simulink model "nxtmouse_ctrl"  (Simulink 6.4)
settings: Solver=FixedStepDiscrete  SolverMode=SingleTasking  StartTime=0  StopTime=inf  FixedStep=0.001  RelTol=1e-3
PreLoadFcn:
  | param;
libraries: ecrobot_nxt_lib x13
CloseFcn:
  | rtwprivate ssgencode ModelCloseRequest nxtcar_ctrl
settings Model: Creator=tchikama  LastModifiedBy=tchikama  ProdHWDeviceType=ARM7
settings DataIOCC: LimitDataPoints=off  SaveOutput=off  SignalLogging=off  SaveTime=off
settings OptimizationCC: InlineParams=on  InlineInvariantSignals=on  RollThreshold=2  StateBitsets=on  DataBitsets=on  UseTempVars=on  InitFltsAndDblsToZero=off  NoFixptDivByZeroProtection=on  EfficientFloat2IntCast=on  OptimizeModelRefInitCode=on  LifeSpan=1
settings DebuggingCC: ConsistencyChecking=warning  SignalInfNanChecking=warning  ReadBeforeWriteMsg=DisableAll  WriteAfterWriteMsg=DisableAll  WriteAfterReadMsg=DisableAll  AlgebraicLoopMsg=error  CheckExecutionContextPreStartOutputMsg=on  CheckExecutionContextRuntimeOutputMsg=on  SolverPrmCheckMsg=none  SingleTaskRateTransMsg=warning  TasksWithSamePriorityMsg=none  IntegerOverflowMsg=error  ParameterUnderflowMsg=warning  ParameterPrecisionLossMsg=none  UnconnectedInputMsg=error  UnconnectedOutputMsg=error  UnconnectedLineMsg=error  UniqueDataStoreMsg=error  BusObjectLabelMismatch=error  RootOutportRequireBusObject=error  ModelReferenceIOMsg=warning  ModelReferenceVersionMismatchMessage=warning  ModelReferenceIOMismatchMessage=warning
settings HardwareCC: ProdIntDivRoundTo=Zero  ProdEndianess=LittleEndian  ProdHWDeviceType=ARM7  TargetHWDeviceType=32-bit Generic
settings ModelReferenceCC: ModelReferenceNumInstancesAllowed=Single
settings RTWCC: SystemTargetFile=ert.tlc  GenCodeOnly=on  GenerateMakefile=off  TemplateMakefile=ert_default_tmf  Description=Real-Time Workshop Embedded Coder (no auto configuration)  GenerateReport=on  RTWVerbose=off  ProcessScript=ert_make_rtw_hook  IncludeHyperlinkInReport=on  LaunchReport=on
settings CodeAppCC: ForceParamTrailComments=on  IgnoreCustomStorageClasses=off  SFDataObjDesc=on  PrefixModelToSubsysFcnNames=off  CustomSymbolStrGlobalVar=rt$N$M  CustomSymbolStrType=$N$M  CustomSymbolStrFcn=$N$M$F  CustomSymbolStrMacro=$N$M  InsertBlockDesc=on
settings ERTTargetCC: TargetFcnLib=ansi_tfl_tmw.mat  GenFloatMathFcnCalls=GNU  IncludeMdlTerminateFcn=off  SuppressErrorStatus=on  IncludeERTFirstTime=on  SupportAbsoluteTime=off  SupportNonFinite=off  SupportComplex=off  PurelyIntegerCode=on  InlinedParameterPlacement=NonHierarchical  RootIOFormat=Structure reference  ERTCustomFileTemplate=example_file_process.tlc  InitialValueSource=Model

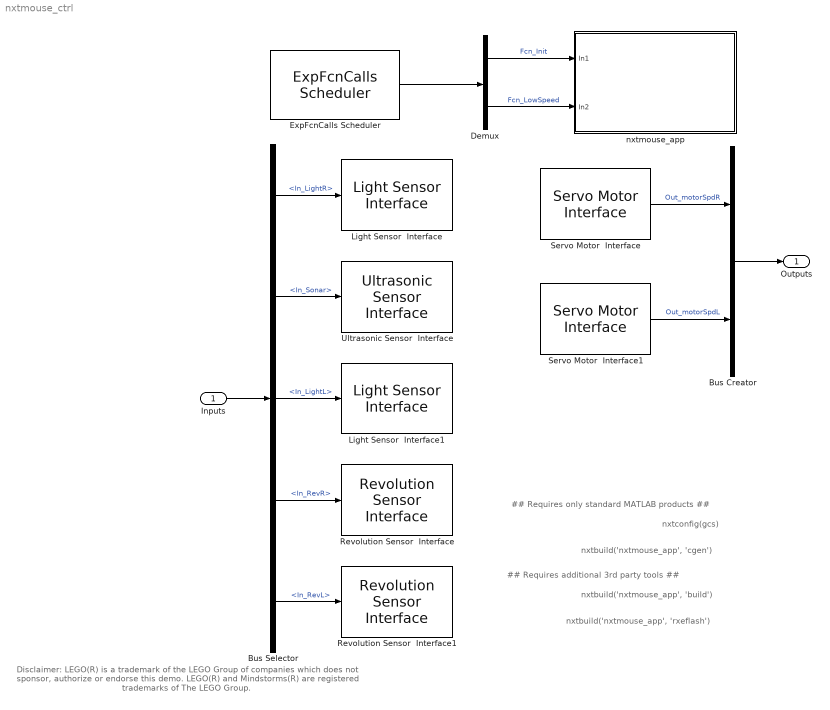
== system nxtmouse_ctrl ==
  note: nxtbuild('nxtmouse_app', 'cgen')
  note: nxtconfig(gcs)
  note: Disclaimer:
      | LEGO(R) is a trademark of the LEGO Group of companies which does not sponsor, authorize or endorse this demo.
      | LEGO(R) and Mindstorms(R)  are registered trademarks of The LEGO Group.
  note: nxtbuild('nxtmouse_app', 'build')
  note: nxtbuild('nxtmouse_app', 'rxeflash')
  note: ## Requires only standard MATLAB products ##
  note: ## Requires additional 3rd party tools ##
  Inputs : Inport  UseBusObject=on
      settings: BusObject=Inputs
  Bus Creator : BusCreator  Inputs=2  UseBusObject=on
      settings: BusObject=Outputs
  Bus Selector : BusSelector  OutputSignals=In_LightR,In_Sonar,In_LightL,In_RevR,In_RevL
  Demux : Demux  Outputs=2
  ExpFcnCalls Scheduler : ecrobot_nxt_lib/ExpFcnCalls Scheduler  Priority=50  fcname='Fcn_Init', 'Fcn_LowSpeed'  fctrigger=[0 50]  ts=0.001  platform=OSEK  stacksize=[512 512]  bd_mode=Slave
  Light Sensor  Interface : ecrobot_nxt_lib/Light Sensor Interface  Priority=0  SystemSampleTime=-1  ip=S2
  Light Sensor  Interface1 : ecrobot_nxt_lib/Light Sensor Interface  Priority=2  SystemSampleTime=-1  ip=S3
  Revolution Sensor  Interface : ecrobot_nxt_lib/Revolution Sensor Interface  Priority=3  SystemSampleTime=-1  ip=B
  Revolution Sensor  Interface1 : ecrobot_nxt_lib/Revolution Sensor Interface  Priority=4  SystemSampleTime=-1  ip=C
  Servo Motor  Interface : ecrobot_nxt_lib/Servo Motor Interface  Priority=100  SystemSampleTime=-1  ip=B  mode=Brake
  Servo Motor  Interface1 : ecrobot_nxt_lib/Servo Motor Interface  Priority=101  SystemSampleTime=-1  ip=C  mode=Brake
  Ultrasonic Sensor  Interface : ecrobot_nxt_lib/Ultrasonic Sensor Interface  Priority=1  SystemSampleTime=-1  ip=S1
  nxtmouse_app : Subsystem
  Outputs : Outport  UseBusObject=on
      settings: BusObject=Outputs
  wires:
  Bus Selector/4 -> Revolution Sensor  Interface/1  "<In_RevR>"
  Bus Selector/5 -> Revolution Sensor  Interface1/1  "<In_RevL>"
  Bus Creator/1 -> Outputs/1
  Inputs/1 -> Bus Selector/1
  Servo Motor  Interface/1 -> Bus Creator/1  "Out_motorSpdR"
  Servo Motor  Interface1/1 -> Bus Creator/2  "Out_motorSpdL"
  ExpFcnCalls Scheduler/1 -> Demux/1
  Demux/1 -> nxtmouse_app/1(In1)  "Fcn_Init"
  Demux/2 -> nxtmouse_app/2(In2)  "Fcn_LowSpeed"
  Bus Selector/2 -> Ultrasonic Sensor  Interface/1  "<In_Sonar>"
  Bus Selector/1 -> Light Sensor  Interface/1  "<In_LightR>"
  Bus Selector/3 -> Light Sensor  Interface1/1  "<In_LightL>"

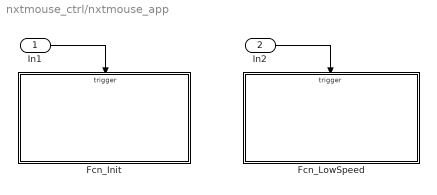
== system nxtmouse_ctrl/nxtmouse_app ==
  In1 : Inport
  In2 : Inport  Port=2
  Fcn_Init : Subsystem  TreatAsAtomicUnit=on
  Fcn_LowSpeed : Subsystem  TreatAsAtomicUnit=on
  wires:
  In1/1 -> Fcn_Init/Trigger
  In2/1 -> Fcn_LowSpeed/Trigger

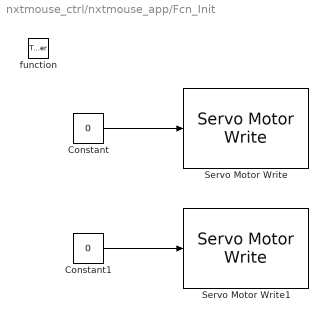
== system nxtmouse_ctrl/nxtmouse_app/Fcn_Init ==
  function : TriggerPort  TriggerType=function-call
  Constant : Constant  Value=0  OutDataType=sfix(16)  ConRadixGroup=Use specified scaling  OutScaling=2^0  SampleTime=inf  FramePeriod=inf
  Constant1 : Constant  Value=0  OutDataType=sfix(16)  ConRadixGroup=Use specified scaling  OutScaling=2^0  SampleTime=inf  FramePeriod=inf
  Servo Motor Write : ecrobot_nxt_lib/Servo Motor Write  SystemSampleTime=-1  ip=B
  Servo Motor Write1 : ecrobot_nxt_lib/Servo Motor Write  SystemSampleTime=-1  ip=C
  wires:
  Constant/1 -> Servo Motor Write/1
  Constant1/1 -> Servo Motor Write1/1

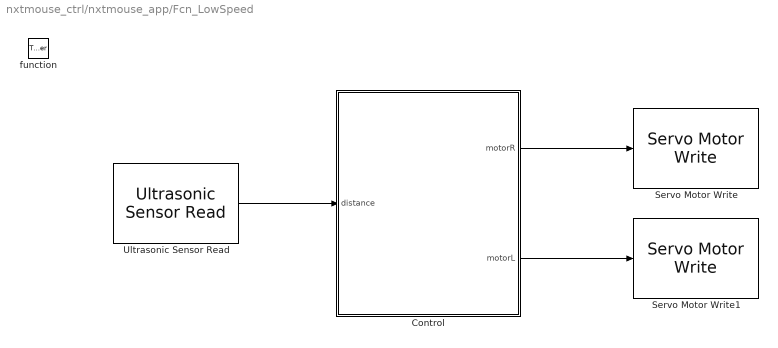
== system nxtmouse_ctrl/nxtmouse_app/Fcn_LowSpeed ==
  function : TriggerPort  TriggerType=function-call
  Control : Stateflow chart  TreatAsAtomicUnit=on
  Servo Motor Write : ecrobot_nxt_lib/Servo Motor Write  SystemSampleTime=-1  ip=B
  Servo Motor Write1 : ecrobot_nxt_lib/Servo Motor Write  SystemSampleTime=-1  ip=C
  Ultrasonic Sensor Read : ecrobot_nxt_lib/Ultrasonic Sensor Read  SystemSampleTime=-1  ip=S1
  wires:
  Control/1(motorR) -> Servo Motor Write/1
  Control/2(motorL) -> Servo Motor Write1/1
  Ultrasonic Sensor Read/1 -> Control/1(distance)

== stateflow chart nxtmouse_app/Fcn_LowSpeed/Control ==
  settings: executeAtInitialization=1
  state forward/
    entry:
    motorR = 100;
    motorL = 100;
  state turn_right/
    entry:
    motorR = -70;
    motorL = 70;
    waitcount=0;
    during: waitcount++;
  state turn_left/
    entry:
    motorR = 70;
    motorL = -70;
    waitcount=0;
    during: waitcount++;
  state backwards/
    entry:
    motorR = -100;
    motorL = -100;
    waitcount=0;
    during: waitcount++;
  (default) -> forward : {t_dir = 2;}
  turn_left -> forward : [waitcount>=6]
      | {t_dir = 1;}
  forward -> backwards : [distance <= 7]
  turn_right -> forward : [waitcount >=6]
      | {t_dir = 2;}
  backwards -> turn_right [order 1] : [waitcount>= 2 && t_dir==1]
  backwards -> turn_left [order 2] : [waitcount>= 2 && t_dir==2]
  data: distance input inherited; motorR output int8; motorL output int8; timer local uint16; t_dir local uint8; waitcount local uint16 =0
  data t_dir settings: description=|
      | touch direction:
      | left sensor = 1, right sensor = 2
